simulink model "rootlocusckt"  (Simulink 7.1)
settings: Solver=ode45  StartTime=0.0  StopTime=10.0  RelTol=1e-3
settings Model: Creator=CARLOS BRUNO  LastModifiedBy=CARLOS BRUNO

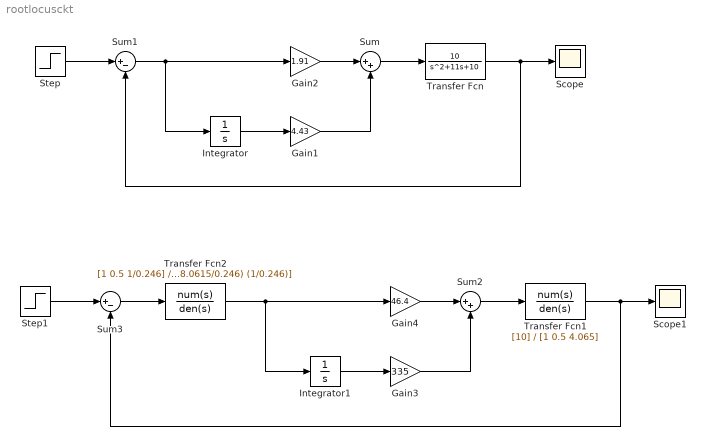
== system rootlocusckt ==
  Gain1 : Gain  Gain=4.43  ParameterDataType=sfix(16)  ParameterScaling=2^0  OutDataType=sfix(16)  OutScaling=2^0
  Gain2 : Gain  Gain=1.91  ParameterDataType=sfix(16)  ParameterScaling=2^0  OutDataType=sfix(16)  OutScaling=2^0
  Gain3 : Gain  Gain=335  ParameterDataType=sfix(16)  ParameterScaling=2^0  OutDataType=sfix(16)  OutScaling=2^0
  Gain4 : Gain  Gain=46.4  ParameterDataType=sfix(16)  ParameterScaling=2^0  OutDataType=sfix(16)  OutScaling=2^0
  Integrator : Integrator
  Integrator1 : Integrator
  Scope : Scope
  Scope1 : Scope
      settings: TimeRange=10
  Step : Step  Time=0  SampleTime=0
  Step1 : Step  Time=0  SampleTime=0
  Sum : Sum  Inputs=|++  OutDataType=sfix(16)  OutScaling=2^0
  Sum1 : Sum  Inputs=|+-  OutDataType=sfix(16)  OutScaling=2^0
  Sum2 : Sum  Inputs=|++  OutDataType=sfix(16)  OutScaling=2^0
  Sum3 : Sum  Inputs=|+-  OutDataType=sfix(16)  OutScaling=2^0
  Transfer Fcn : TransferFcn  Numerator=[10]  Denominator=[1 11 10]
  Transfer Fcn1 : TransferFcn  Numerator=[10]  Denominator=[1 0.5 4.065]
  Transfer Fcn2 : TransferFcn  Numerator=[1 0.5 1/0.246]  Denominator=[1 (8.0615/0.246) (1/0.246)]
  wires:
  Sum/1 -> Transfer Fcn/1
  Gain2/1 -> Sum/1
  Gain1/1 -> Sum/2
  Integrator/1 -> Gain1/1
  Sum1/1 -> Integrator/1, Gain2/1
  Transfer Fcn/1 -> Sum1/2, Scope/1
  Step/1 -> Sum1/1
  Sum2/1 -> Transfer Fcn1/1
  Gain4/1 -> Sum2/1
  Gain3/1 -> Sum2/2
  Integrator1/1 -> Gain3/1
  Transfer Fcn1/1 -> Sum3/2, Scope1/1
  Step1/1 -> Sum3/1
  Transfer Fcn2/1 -> Gain4/1, Integrator1/1
  Sum3/1 -> Transfer Fcn2/1
